simulink model "Aula7"  (R2013b)
settings: Solver=ode45  StartTime=0.0  StopTime=0.3  RelTol=1e-3
libraries: simulink x1
settings Model: Creator=ThiagoCordeiro  LastModifiedBy=ThiagoFelippe

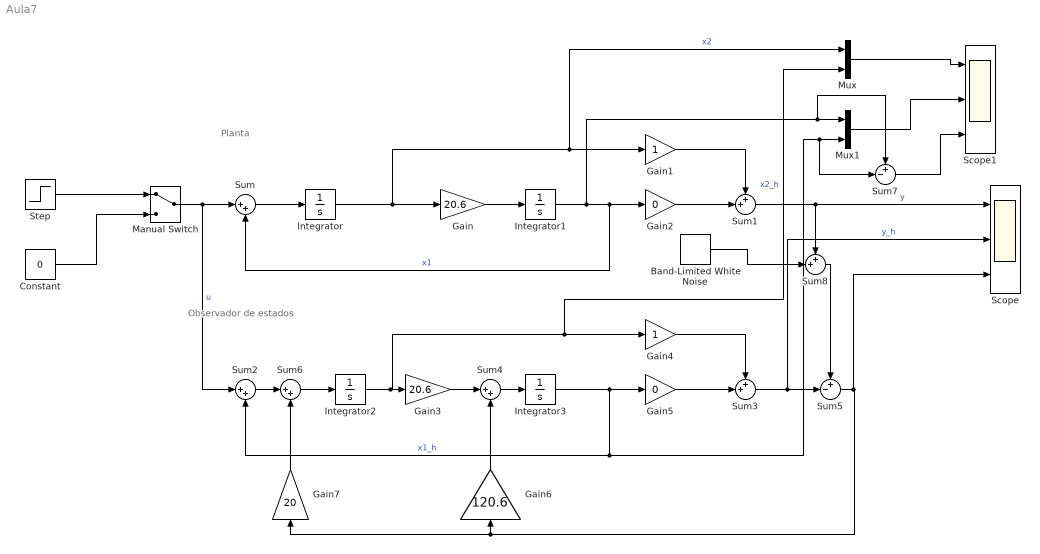
== system Aula7 ==
  note: Planta
  note: Observador de estados
  Band-Limited White Noise : simulink/Sources/Band-Limited White Noise  Cov=[0.01]  Ts=0.01  seed=[23341]
  Constant : Constant  Value=0
  Gain : Gain  Gain=20.6
  Gain1 : Gain
  Gain2 : Gain  Gain=0
  Gain3 : Gain  Gain=20.6
  Gain4 : Gain
  Gain5 : Gain  Gain=0
  Gain6 : Gain  Gain=120.6
  Gain7 : Gain  Gain=20
  Integrator : Integrator  InitialCondition=5
  Integrator1 : Integrator  InitialCondition=1
  Integrator2 : Integrator
  Integrator3 : Integrator
  Manual Switch : ManualSwitch
  Mux : Mux  Inputs=2
  Mux1 : Mux  Inputs=2
  Scope : Scope  NumInputPorts=3
      settings: YMin=-5~-5~-5  YMax=5~5~5
  Scope1 : Scope  NumInputPorts=3
      settings: YMin=-5~-5~-5  YMax=5~5~5
  Step : Step  Time=0.5  SampleTime=0
  Sum{,2,4,6} (4 alike) : Sum  Inputs=|++
  Sum1 : Sum  Inputs=++|
  Sum3 : Sum  Inputs=++|
  Sum5 : Sum  Inputs=+-|
  Sum7 : Sum  Inputs=+-|
  Sum8 : Sum  Inputs=++|
  wires:
  Step/1 -> Manual Switch/1
  Sum/1 -> Integrator/1
  Constant/1 -> Manual Switch/2
  Integrator/1 -> Mux/1, Gain1/1, Gain/1  "x2"
  Gain/1 -> Integrator1/1
  Integrator1/1 -> Sum7/1, Mux1/1, Sum/2, Gain2/1  "x1"
  Gain2/1 -> Sum1/2
  Gain1/1 -> Sum1/1
  Sum1/1 -> Scope/1, Sum8/1  "y"
  Manual Switch/1 -> Sum2/1, Sum/1  "u"
  Integrator2/1 -> Mux/2, Gain4/1, Gain3/1  "x2_h"
  Integrator3/1 -> Gain5/1, Sum7/2, Mux1/2, Sum2/2  "x1_h"
  Gain5/1 -> Sum3/2
  Gain4/1 -> Sum3/1
  Sum3/1 -> Scope/2, Sum5/2  "y_h"
  Gain3/1 -> Sum4/1
  Sum4/1 -> Integrator3/1
  Gain6/1 -> Sum4/2
  Sum5/1 -> Scope/3, Gain7/1, Gain6/1
  Sum2/1 -> Sum6/1
  Sum6/1 -> Integrator2/1
  Gain7/1 -> Sum6/2
  Mux/1 -> Scope1/1
  Mux1/1 -> Scope1/2
  Sum7/1 -> Scope1/3
  Band-Limited White Noise/1 -> Sum8/2
  Sum8/1 -> Sum5/1
